simulink model "test2"  (R2014b)
settings: Solver=ode45  StartTime=0.0  StopTime=5  MaxStep=0.0001  RelTol=1e-3
libraries: simulink x1, fuzblock x1, powerlib x1
settings Model: Creator=Administrator  LastModifiedBy=Administrator
settings SolverCC: ZeroCrossControl=DisableAll

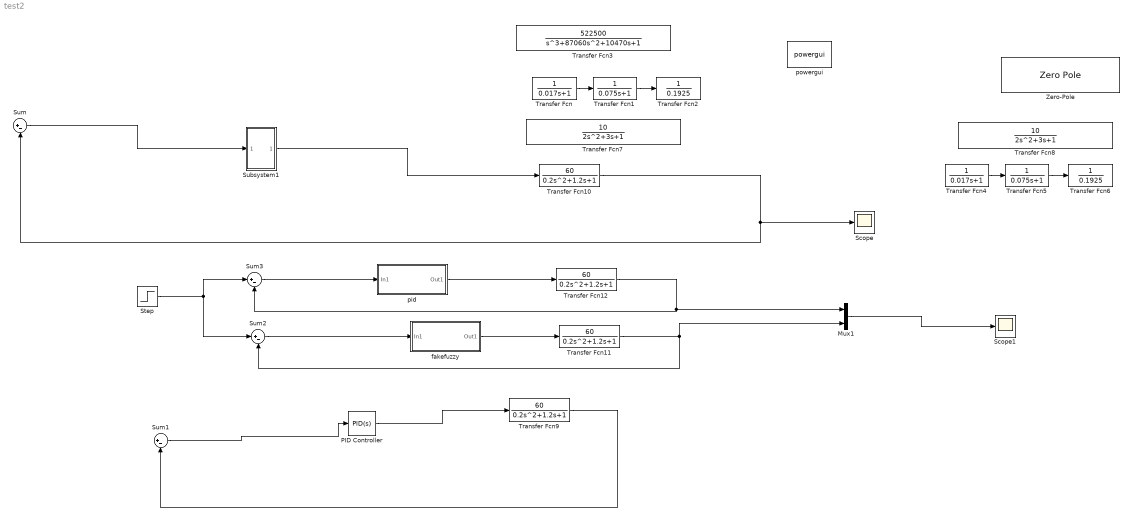
== system test2 ==
  Mux1 : Mux  Inputs=2
  PID Controller : simulink/Continuous/PID Controller  Controller=PID  TimeDomain=Continuous-time  SampleTime=-1  IntegratorMethod=Forward Euler  FilterMethod=Forward Euler  Form=Parallel  P=0.117282940590111  I=0.100100462071738  D=0.0111808329497982  N=15.1755472667856  InitialConditionSource=internal  InitialConditionForIntegrator=0  InitialConditionForFilter=0  ExternalReset=none  LimitOutput=off  UpperSaturationLimit=inf  LowerSaturationLimit=-inf  LinearizeAsGain=on  AntiWindupMode=none  Kb=1  TrackingMode=off  Kt=1  PParamMin=[]  PParamMax=[]  IParamMin=[]  IParamMax=[]  DParamMin=[]  DParamMax=[]  NParamMin=[]  NParamMax=[]  KbParamMin=[]  KbParamMax=[]  KtParamMin=[]  KtParamMax=[]  POutMin=[]  POutMax=[]  IOutMin=[]  IOutMax=[]  DOutMin=[]  DOutMax=[]  NOutMin=[]  NOutMax=[]  KbOutMin=[]  KbOutMax=[]  KtOutMin=[]  KtOutMax=[]  IntegratorOutMin=[]  IntegratorOutMax=[]  FilterOutMin=[]  FilterOutMax=[]  SumOutMin=[]  SumOutMax=[]  SumI1OutMin=[]  SumI1OutMax=[]  SumI2OutMin=[]  SumI2OutMax=[]  SumI3OutMin=[]  SumI3OutMax=[]  SumDOutMin=[]  SumDOutMax=[]  SaturationOutMin=[]  SaturationOutMax=[]  IntegratorContinuousStateAttributes=''  IntegratorStateMustResolveToSignalObject=off  IntegratorRTWStateStorageClass=Auto  FilterContinuousStateAttributes=''  FilterStateMustResolveToSignalObject=off  FilterRTWStateStorageClass=Auto  DifferentiatorICPrevScaledInput=0  DifferentiatorOutMin=[]  DifferentiatorOutMax=[]  UseFilter=on
  Scope : Scope
      settings: YMin=-1.4e+130  YMax=4e+129
  Scope1 : Scope
      settings: YMin=0  YMax=60
  Step : Step  After=50  SampleTime=0
  Subsystem1 : Subsystem
  Sum{,1..3} (4 alike) : Sum  Inputs=|+-
  Transfer Fcn : TransferFcn  Denominator=[0.017 1]
  Transfer Fcn1 : TransferFcn  Denominator=[0.075 1]
  Transfer Fcn{9..12} (4 alike) : TransferFcn  Numerator=[60]  Denominator=[0.2 1.2 1]
  Transfer Fcn2 : TransferFcn  Denominator=[0.1925]
  Transfer Fcn3 : TransferFcn  Numerator=[522500]  Denominator=[1 87060 10470 1]
  Transfer Fcn4 : TransferFcn  Denominator=[0.017 1]
  Transfer Fcn5 : TransferFcn  Denominator=[0.075 1]
  Transfer Fcn6 : TransferFcn  Denominator=[0.1925]
  Transfer Fcn7 : TransferFcn  Numerator=[10]  Denominator=[2 3 1]
  Transfer Fcn8 : TransferFcn  Numerator=[10]  Denominator=[2 3 1]
  Zero-Pole : ZeroPole  Zeros=[-0.5]  Poles=[-1 -1 -1]  Gain=[10]
  fakefuzzy : Subsystem
  pid : Subsystem
  powergui : powerlib/powergui  Priority=1  SimulationMode=Continuous  SolverType=Tustin/Backward Euler (TBE)  SampleTime=50e-6  frequency=60  SPID=off  DisableSnubberDevices=off  DisableRonSwitches=off  DisableVfSwitches=off  SwTol=0  DisplayEquations=off  Interpol=off  methode=off  Ts=100  frequencyindice=60  Pbase=100e6  ErrMax=1e-4  Iterations=50  UnitsV=kV  UnitsW=MW  FunctionMessages=off  echomessages=off  HookPort=off  EnableUseOfTLC=off  x0status=blocks  RestoreLinks=warning  ResistiveCurrentMeasurement=off  Frange=[0:2:500]  Ylog=off  Xlog=on  ShowGrid=off  save=off  variable=ZData  structure=0  ZoomFFT=off  StartTime=0.0  cycles=1  DisplayStyle=1  fundamental=60  FreqAxis=off  MaxFrequency=1000  frequencyindicesteady=1  RmsSteady=1  display=off
  wires:
  Transfer Fcn/1 -> Transfer Fcn1/1
  Transfer Fcn1/1 -> Transfer Fcn2/1
  Transfer Fcn4/1 -> Transfer Fcn5/1
  Transfer Fcn5/1 -> Transfer Fcn6/1
  Sum1/1 -> PID Controller/1
  Transfer Fcn9/1 -> Sum1/2
  PID Controller/1 -> Transfer Fcn9/1
  Transfer Fcn10/1 -> Sum/2, Scope/1
  fakefuzzy/1(Out1) -> Transfer Fcn11/1
  Mux1/1 -> Scope1/1
  Transfer Fcn11/1 -> Sum2/2, Mux1/2
  Sum2/1 -> fakefuzzy/1(In1)
  Transfer Fcn12/1 -> Mux1/1, Sum3/2
  Sum3/1 -> pid/1(In1)
  pid/1(Out1) -> Transfer Fcn12/1
  Step/1 -> Sum3/1, Sum2/1
  Sum/1 -> Subsystem1/1(In1)
  Subsystem1/1(Out1) -> Transfer Fcn10/1

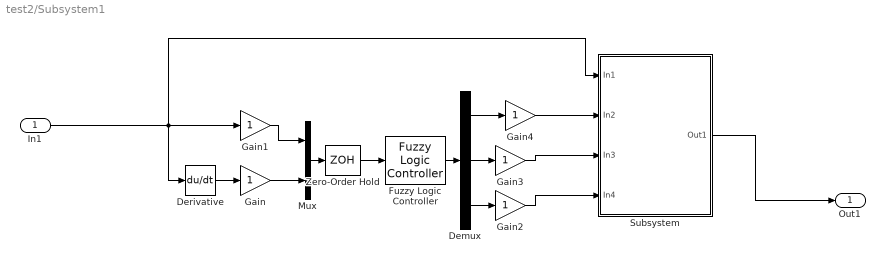
== system test2/Subsystem1 ==
  In1 : Inport
  Demux : Demux  Outputs=3
  Derivative : Derivative
  Fuzzy Logic Controller : fuzblock/Fuzzy Logic  Controller  fis=fuzzy_1
  Gain{,1..4} (5 alike) : Gain
  Mux : Mux  Inputs=2
  Subsystem : Subsystem
  Zero-Order Hold : ZeroOrderHold
  Out1 : Outport
  wires:
  Fuzzy Logic Controller/1 -> Demux/1
  Mux/1 -> Zero-Order Hold/1
  Derivative/1 -> Gain/1
  In1/1 -> Derivative/1, Gain1/1, Subsystem/1(In1)
  Zero-Order Hold/1 -> Fuzzy Logic Controller/1
  Demux/1 -> Gain4/1
  Demux/2 -> Gain3/1
  Demux/3 -> Gain2/1
  Gain4/1 -> Subsystem/2(In2)
  Gain3/1 -> Subsystem/3(In3)
  Gain2/1 -> Subsystem/4(In4)
  Gain1/1 -> Mux/1
  Gain/1 -> Mux/2
  Subsystem/1(Out1) -> Out1/1

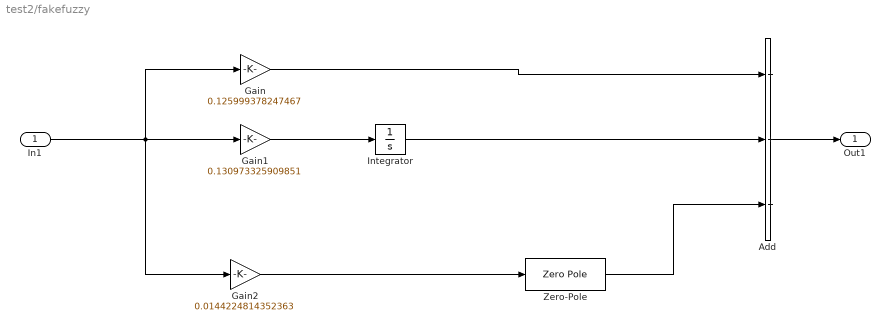
== system test2/fakefuzzy ==
  In1 : Inport
  Add : Sum  Inputs=+++
  Gain : Gain  Gain=0.125999378247467
  Gain1 : Gain  Gain=0.130973325909851
  Gain2 : Gain  Gain=0.0144224814352363
  Integrator : Integrator
  Zero-Pole : ZeroPole  Zeros=[0]  Poles=[-32.0224147617823]  Gain=[32.0224147617823]
  Out1 : Outport
  wires:
  Add/1 -> Out1/1
  Gain1/1 -> Integrator/1
  Integrator/1 -> Add/2
  In1/1 -> Gain2/1, Gain/1, Gain1/1
  Gain/1 -> Add/1
  Zero-Pole/1 -> Add/3
  Gain2/1 -> Zero-Pole/1

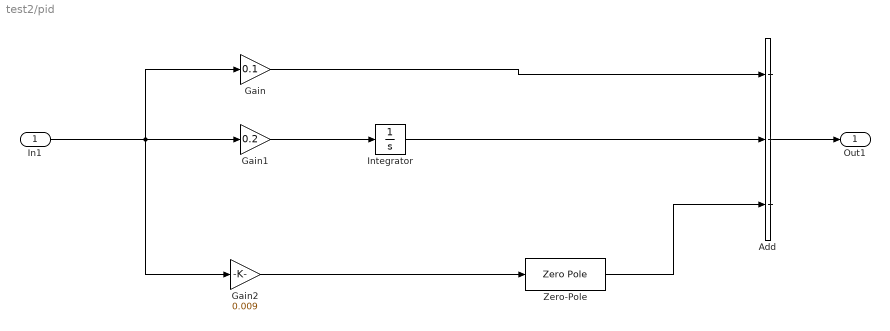
== system test2/pid ==
  In1 : Inport
  Add : Sum  Inputs=+++
  Gain : Gain  Gain=0.1
  Gain1 : Gain  Gain=0.2
  Gain2 : Gain  Gain=0.009
  Integrator : Integrator
  Zero-Pole : ZeroPole  Zeros=[0]  Poles=[-32.0224147617823]  Gain=[32.0224147617823]
  Out1 : Outport
  wires:
  Add/1 -> Out1/1
  Gain1/1 -> Integrator/1
  Integrator/1 -> Add/2
  In1/1 -> Gain2/1, Gain/1, Gain1/1
  Gain/1 -> Add/1
  Zero-Pole/1 -> Add/3
  Gain2/1 -> Zero-Pole/1

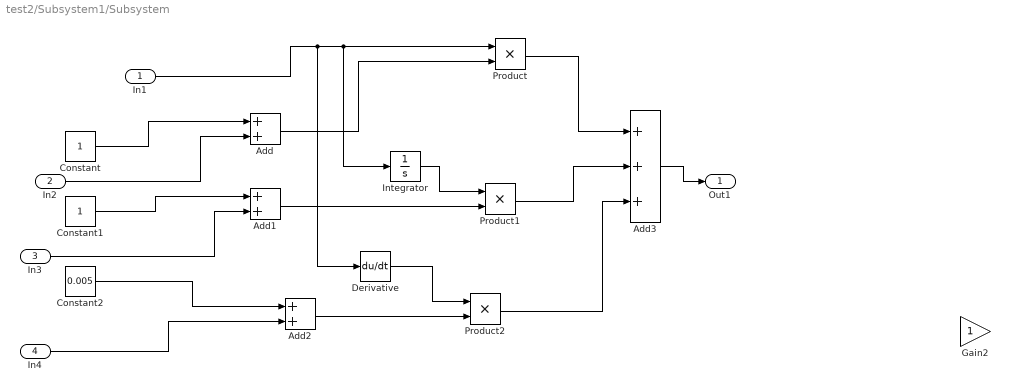
== system test2/Subsystem1/Subsystem ==
  In1 : Inport
  In2 : Inport  Port=2
  In3 : Inport  Port=3
  In4 : Inport  Port=4
  Add : Sum
  Add1 : Sum
  Add2 : Sum
  Add3 : Sum  Inputs=+++
  Constant : Constant
  Constant1 : Constant
  Constant2 : Constant  Value=0.005
  Derivative : Derivative
  Gain2 : Gain
  Integrator : Integrator
  Product : Product
  Product1 : Product
  Product2 : Product
  Out1 : Outport
  wires:
  In1/1 -> Derivative/1, Integrator/1, Product/1
  Add/1 -> Product/2
  Integrator/1 -> Product1/1
  Derivative/1 -> Product2/1
  Add2/1 -> Product2/2
  Add1/1 -> Product1/2
  Product/1 -> Add3/1
  Product1/1 -> Add3/2
  Product2/1 -> Add3/3
  Add3/1 -> Out1/1
  In4/1 -> Add2/2
  In3/1 -> Add1/2
  In2/1 -> Add/2
  Constant/1 -> Add/1
  Constant1/1 -> Add1/1
  Constant2/1 -> Add2/1
